simulink model "SixJointFixTimeMode"  (R2019b)
settings: Solver=ode45  StartTime=0.0  StopTime=1  FixedStep=0.01  RelTol=1e-3
values from neighbouring files (symbols this model uses):
  m = [m1;m2;m3;m4;m5;m6]    [SixJointFiniteTimeController.m]    (also in SixJointFixTimeController.m; SixJointFixTimeController2.m; SixJointFixTimeController3.m; SixJointFixTimePlant.m)
  N = N1+N2+N3+N4+N5+N6    [SixJointFiniteTimeController.m]    (also in SixJointFixTimeController.m; SixJointFixTimeController2.m; SixJointFixTimeController3.m; SixJointFixTimePlant.m)
  s = [s1; s2; s3; s4; s5; s6]    [SixJointFiniteTimeController.m]    (also in ctrl2_nijunkang.m = -de + alpha1*abs(-e)^p*sign(-e) + belta1*abs(-e)^E2*sign(-e); ctrl2_test.m = dth + alpha1*abs(th)^p*sign(th) + belta1*abs(th)^E2*sign(th))
undefined symbols (not defined in the file or in its folder): X, Y, Z
libraries: sm_lib x22, nesl_utility x19
settings Model: Creator=user  LastModifiedBy=xyh
settings SolverCC: AlgebraicLoopSolver=LineSearch
settings DataIOCC: ReturnWorkspaceOutputs=off

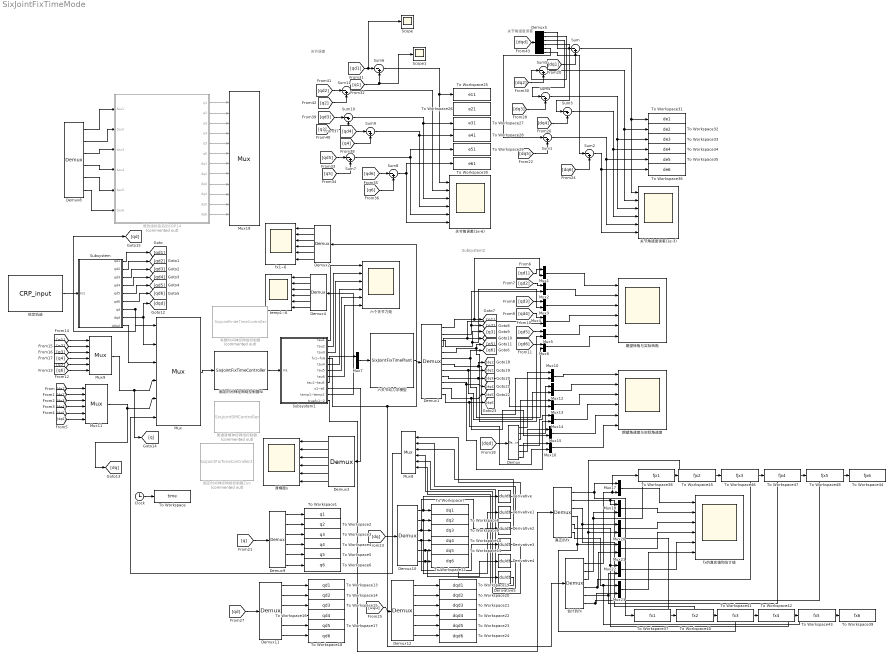
== system SixJointFixTimeMode ==
  note: 关节误差
  note: 关节角速度误差
  note: Subsystem2
  Clock : Clock
  Demux{,2..5,8..12} (10 alike) : Demux  Outputs=6
  Demux1 : Demux  Outputs=12
  Derivative{,1..5} (6 alike) : Derivative
  Mux{,8..9,11} (4 alike) : Mux  Inputs=6
  Mux{1..7,10,12..18,20..23} (19 alike) : Mux  Inputs=2
  Mux19 : Mux  Inputs=12
  Scope : Scope
  Scope1 : Scope
  Subsystem : Subsystem  TreatAsAtomicUnit=on
  Subsystem1 : Subsystem
  Sum{,1..11} (12 alike) : Sum  Inputs=|-+
  To Workspace : ToWorkspace  VariableName=time  SaveFormat=Timeseries  SampleTime=-1
  To Workspace1 : ToWorkspace  VariableName=q1  SaveFormat=Timeseries  SampleTime=-1
  To Workspace10 : ToWorkspace  VariableName=dq4  SaveFormat=Timeseries  SampleTime=-1
  To Workspace11 : ToWorkspace  VariableName=dq5  SaveFormat=Timeseries  SampleTime=-1
  To Workspace12 : ToWorkspace  VariableName=dq6  SaveFormat=Timeseries  SampleTime=-1
  To Workspace13 : ToWorkspace  VariableName=qd1  SaveFormat=Timeseries  SampleTime=-1
  To Workspace14 : ToWorkspace  VariableName=qd2  SaveFormat=Timeseries  SampleTime=-1
  To Workspace15 : ToWorkspace  VariableName=qd3  SaveFormat=Timeseries  SampleTime=-1
  To Workspace16 : ToWorkspace  VariableName=qd4  SaveFormat=Timeseries  SampleTime=-1
  To Workspace17 : ToWorkspace  VariableName=qd5  SaveFormat=Timeseries  SampleTime=-1
  To Workspace18 : ToWorkspace  VariableName=qd6  SaveFormat=Timeseries  SampleTime=-1
  To Workspace19 : ToWorkspace  VariableName=dqd1  SaveFormat=Timeseries  SampleTime=-1
  To Workspace2 : ToWorkspace  VariableName=q2  SaveFormat=Timeseries  SampleTime=-1
  To Workspace20 : ToWorkspace  VariableName=dqd2  SaveFormat=Timeseries  SampleTime=-1
  To Workspace21 : ToWorkspace  VariableName=dqd3  SaveFormat=Timeseries  SampleTime=-1
  To Workspace22 : ToWorkspace  VariableName=dqd4  SaveFormat=Timeseries  SampleTime=-1
  To Workspace23 : ToWorkspace  VariableName=dqd5  SaveFormat=Timeseries  SampleTime=-1
  To Workspace24 : ToWorkspace  VariableName=dqd6  SaveFormat=Timeseries  SampleTime=-1
  To Workspace25 : ToWorkspace  VariableName=e11  SaveFormat=Timeseries  SampleTime=-1
  To Workspace26 : ToWorkspace  VariableName=e21  SaveFormat=Timeseries  SampleTime=-1
  To Workspace27 : ToWorkspace  VariableName=e31  SaveFormat=Timeseries  SampleTime=-1
  To Workspace28 : ToWorkspace  VariableName=e41  SaveFormat=Timeseries  SampleTime=-1
  To Workspace29 : ToWorkspace  VariableName=e51  SaveFormat=Timeseries  SampleTime=-1
  To Workspace3 : ToWorkspace  VariableName=q3  SaveFormat=Timeseries  SampleTime=-1
  To Workspace30 : ToWorkspace  VariableName=e61  SaveFormat=Timeseries  SampleTime=-1
  To Workspace31 : ToWorkspace  VariableName=de1  SaveFormat=Timeseries  SampleTime=-1
  To Workspace32 : ToWorkspace  VariableName=de2  SaveFormat=Timeseries  SampleTime=-1
  To Workspace33 : ToWorkspace  VariableName=de3  SaveFormat=Timeseries  SampleTime=-1
  To Workspace34 : ToWorkspace  VariableName=de4  SaveFormat=Timeseries  SampleTime=-1
  To Workspace35 : ToWorkspace  VariableName=de5  SaveFormat=Timeseries  SampleTime=-1
  To Workspace36 : ToWorkspace  VariableName=de6  SaveFormat=Timeseries  SampleTime=-1
  To Workspace37 : ToWorkspace  VariableName=fx1  SaveFormat=Timeseries  SampleTime=-1
  To Workspace38 : ToWorkspace  VariableName=fjx1  SaveFormat=Timeseries  SampleTime=-1
  To Workspace39 : ToWorkspace  VariableName=fx6  SaveFormat=Timeseries  SampleTime=-1
  To Workspace4 : ToWorkspace  VariableName=q4  SaveFormat=Timeseries  SampleTime=-1
  To Workspace40 : ToWorkspace  VariableName=fx2  SaveFormat=Timeseries  SampleTime=-1
  To Workspace41 : ToWorkspace  VariableName=fx3  SaveFormat=Timeseries  SampleTime=-1
  To Workspace42 : ToWorkspace  VariableName=fx4  SaveFormat=Timeseries  SampleTime=-1
  To Workspace43 : ToWorkspace  VariableName=fx5  SaveFormat=Timeseries  SampleTime=-1
  To Workspace44 : ToWorkspace  VariableName=fjx6  SaveFormat=Timeseries  SampleTime=-1
  To Workspace45 : ToWorkspace  VariableName=fjx2  SaveFormat=Timeseries  SampleTime=-1
  To Workspace46 : ToWorkspace  VariableName=fjx3  SaveFormat=Timeseries  SampleTime=-1
  To Workspace47 : ToWorkspace  VariableName=fjx4  SaveFormat=Timeseries  SampleTime=-1
  To Workspace48 : ToWorkspace  VariableName=fjx5  SaveFormat=Timeseries  SampleTime=-1
  To Workspace5 : ToWorkspace  VariableName=q5  SaveFormat=Timeseries  SampleTime=-1
  To Workspace6 : ToWorkspace  VariableName=q6  SaveFormat=Timeseries  SampleTime=-1
  To Workspace7 : ToWorkspace  VariableName=dq1  SaveFormat=Timeseries  SampleTime=-1
  To Workspace8 : ToWorkspace  VariableName=dq2  SaveFormat=Timeseries  SampleTime=-1
  To Workspace9 : ToWorkspace  VariableName=dq3  SaveFormat=Timeseries  SampleTime=-1
  fx1~6 : Scope  NumInputPorts=6
  "fx的真实值和估计值 " : Scope  NumInputPorts=6
  temp1~6 : Scope  NumInputPorts=6
  估计的fx : Demux  Outputs=6
  "修改坐标系后的CRP14 " : Subsystem  Commented=on
      mask Display: image('$imagefile'); % Use "Edit Image" on toolstrip to change.
  六个关节力矩 : Scope  NumInputPorts=6
  "六关节动力学模型 " : S-Function  FunctionName=SixJointFixTimePlant  SFunctionDeploymentMode=off  EnableBusSupport=off
  关节角误差(1e-6) : Scope  NumInputPorts=6
  关节角速度误差(1e-3) : Scope  NumInputPorts=6
  固定时间神经网络控制器Ni : S-Function  FunctionName=SixJointFixTimeController  SFunctionDeploymentMode=off  EnableBusSupport=off
  固定时间神经网络控制器Zuo : S-Function  Commented=on  FunctionName=SixJointFixTimeController2  SFunctionDeploymentMode=off  EnableBusSupport=off
  普通滑模神经网络控制器 : S-Function  Commented=on  FunctionName=SixJointSMController  SFunctionDeploymentMode=off  EnableBusSupport=off
  有限时间神经网络控制器 : S-Function  Commented=on  FunctionName=SixJointFiniteTimeController  SFunctionDeploymentMode=off  EnableBusSupport=off
  期望角速度与实际角速度 : Scope  NumInputPorts=6
  期望转角与实际转角 : Scope  NumInputPorts=6
  滑模面s : Scope  NumInputPorts=6
  真正的fx : Demux  Outputs=6
  给定轨迹 : S-Function  FunctionName=CRP_input  SFunctionDeploymentMode=off  EnableBusSupport=off
  wires:
  Clock/1 -> To Workspace/1
  [dq1] -> Mux11/1
  [dq4] -> Mux11/4
  [dq2] -> Mux11/2
  [dq3] -> Mux11/3
  [dq5] -> Mux11/5
  [dq6] -> Mux11/6
  Demux3/1 -> 滑模面s/1
  Demux3/2 -> 滑模面s/2
  Demux3/3 -> 滑模面s/3
  [q1] -> Mux9/1
  [q2] -> Mux9/2
  [q3] -> Mux9/3
  [q4] -> Mux9/4
  [q5] -> Mux9/5
  [q6] -> Mux9/6
  "六关节动力学模型 "/1 -> Demux1/1
  Mux11/1 -> [dq], Mux/5
  Mux9/1 -> [q], Mux/4
  给定轨迹/1 -> Subsystem/1(In1)
  Subsystem/7(qd) -> [qd], Mux/1
  Subsystem/8(dqd) -> [dqd], Mux/2
  Subsystem/9(ddqd) -> Mux/3
  Subsystem/1(qd1) -> [qd1]
  Subsystem/2(qd2) -> [qd2]
  Subsystem/3(qd3) -> [qd3]
  Subsystem/4(qd4) -> [qd4]
  Subsystem/5(qd5) -> [qd5]
  Subsystem/6(qd6) -> [qd6]
  Sum6/1 -> 关节角误差(1e-6)/1, To Workspace25/1
  Sum11/1 -> 关节角误差(1e-6)/2, To Workspace26/1
  Sum10/1 -> 关节角误差(1e-6)/3, To Workspace27/1
  Sum9/1 -> 关节角误差(1e-6)/4, To Workspace28/1
  Sum7/1 -> To Workspace29/1, 关节角误差(1e-6)/5
  Sum8/1 -> 关节角误差(1e-6)/6, To Workspace30/1
  Mux1/1 -> 期望转角与实际转角/1
  Mux2/1 -> 期望转角与实际转角/2
  Mux3/1 -> 期望转角与实际转角/3
  Mux4/1 -> 期望转角与实际转角/4
  Mux5/1 -> 期望转角与实际转角/5
  Mux6/1 -> 期望转角与实际转角/6
  Mux10/1 -> 期望角速度与实际角速度/1
  Mux12/1 -> 期望角速度与实际角速度/2
  Mux13/1 -> 期望角速度与实际角速度/3
  Mux14/1 -> 期望角速度与实际角速度/4
  Mux15/1 -> 期望角速度与实际角速度/5
  Mux16/1 -> 期望角速度与实际角速度/6
  Demux/4 -> Mux14/1
  Demux1/12 -> Mux16/2, [dq6]
  Demux1/2 -> [q2], Mux2/2
  [qd2] -> Mux2/1
  Demux1/4 -> Mux4/2, [q4]
  [qd1] -> Mux1/1
  Demux/3 -> Mux13/1
  Demux/6 -> Mux16/1
  Demux1/10 -> Mux14/2, [dq4]
  Demux/5 -> Mux15/1
  Demux/1 -> Mux10/1
  Demux1/9 -> Mux13/2, [dq3]
  [dqd] -> Demux/1
  [qd6] -> Mux6/1
  Demux1/7 -> Mux10/2, [dq1]
  [qd3] -> Mux3/1
  Demux1/11 -> [dq5], Mux15/2
  [qd4] -> Mux4/1
  [qd5] -> Mux5/1
  Demux1/5 -> Mux5/2, [q5]
  Demux/2 -> Mux12/1
  Demux1/6 -> [q6], Mux6/2
  Demux1/8 -> Mux12/2, [dq2]
  Demux1/3 -> [q3], Mux3/2
  Sum/1 -> To Workspace31/1, 关节角速度误差(1e-3)/1
  Sum5/1 -> To Workspace32/1, 关节角速度误差(1e-3)/2
  Sum4/1 -> To Workspace33/1, 关节角速度误差(1e-3)/3
  Sum3/1 -> 关节角速度误差(1e-3)/4, To Workspace34/1
  Sum1/1 -> 关节角速度误差(1e-3)/5, To Workspace35/1
  Sum2/1 -> 关节角速度误差(1e-3)/6, To Workspace36/1
  [dq2] -> Sum5/2
  Demux5/4 -> Sum3/1
  Demux5/5 -> Sum1/1
  Demux5/3 -> Sum4/1
  [dq5] -> Sum1/2
  Demux5/1 -> Sum/1
  [dq6] -> Sum2/2
  Demux5/6 -> Sum2/1
  Demux5/2 -> Sum5/1
  [dq3] -> Sum4/2
  [dq4] -> Sum3/2
  [dq1] -> Sum/2
  [q5] -> Sum7/2
  [qd1] -> Scope/1, Sum6/1
  [qd2] -> Sum11/1
  [q4] -> Sum9/2
  [qd3] -> Sum10/1
  [qd4] -> Sum9/1
  [q3] -> Sum10/2
  [qd5] -> Sum7/1
  [q6] -> Sum8/2
  [qd6] -> Sum8/1
  [q2] -> Sum11/2
  [q1] -> Scope1/1, Sum6/2
  [dqd] -> Demux5/1
  Mux/1 -> 固定时间神经网络控制器Ni/1
  Demux3/4 -> 滑模面s/4
  Demux3/5 -> 滑模面s/5
  Demux3/6 -> 滑模面s/6
  Demux2/1 -> fx1~6/1
  Demux2/2 -> fx1~6/2
  Demux2/3 -> fx1~6/3
  Demux2/4 -> fx1~6/4
  Demux2/5 -> fx1~6/5
  Demux2/6 -> fx1~6/6
  "修改坐标系后的CRP14 "/1(q1) -> Mux19/1
  "修改坐标系后的CRP14 "/2(q2) -> Mux19/2
  "修改坐标系后的CRP14 "/3(q3) -> Mux19/3
  "修改坐标系后的CRP14 "/4(q4) -> Mux19/4
  "修改坐标系后的CRP14 "/5(q5) -> Mux19/5
  "修改坐标系后的CRP14 "/6(q6) -> Mux19/6
  "修改坐标系后的CRP14 "/7(dq1) -> Mux19/7
  "修改坐标系后的CRP14 "/8(dq2) -> Mux19/8
  "修改坐标系后的CRP14 "/9(dq3) -> Mux19/9
  "修改坐标系后的CRP14 "/10(dq4) -> Mux19/10
  "修改坐标系后的CRP14 "/11(dq5) -> Mux19/11
  "修改坐标系后的CRP14 "/12(dq6) -> Mux19/12
  Demux8/1 -> "修改坐标系后的CRP14 "/1(tau1)
  Demux8/2 -> "修改坐标系后的CRP14 "/2(tau2)
  Demux8/3 -> "修改坐标系后的CRP14 "/3(tau3)
  Demux8/4 -> "修改坐标系后的CRP14 "/4(tau4)
  Demux8/5 -> "修改坐标系后的CRP14 "/5(tau5)
  Demux8/6 -> "修改坐标系后的CRP14 "/6(tau6)
  固定时间神经网络控制器Ni/1 -> Subsystem1/1(In1)
  Subsystem1/1(tau1) -> 六个关节力矩/1
  Subsystem1/2(tau2) -> 六个关节力矩/2
  Subsystem1/3(tau3) -> 六个关节力矩/3
  Subsystem1/5(tau4) -> 六个关节力矩/4
  Subsystem1/6(tau5) -> 六个关节力矩/5
  Subsystem1/7(tau6) -> 六个关节力矩/6
  Subsystem1/9(s1~s6) -> Demux3/1
  Subsystem1/4(fx1~fx6) -> Demux2/1, 估计的fx/1
  Subsystem1/8(tau1~tau6) -> Mux7/1
  Demux4/6 -> temp1~6/6
  Demux4/5 -> temp1~6/5
  Demux4/4 -> temp1~6/4
  Demux4/3 -> temp1~6/3
  Demux4/2 -> temp1~6/2
  Demux4/1 -> temp1~6/1
  Subsystem1/10(temp1~temp1) -> Demux4/1
  Mux7/1 -> "六关节动力学模型 "/1
  [q] -> Demux9/1
  [dq] -> Demux10/1
  [qd] -> Demux11/1
  [dqd] -> Demux12/1
  Demux11/1 -> To Workspace13/1
  Demux11/2 -> To Workspace14/1
  Demux11/3 -> To Workspace15/1
  Demux11/4 -> To Workspace16/1
  Demux11/5 -> To Workspace17/1
  Demux11/6 -> To Workspace18/1
  Demux12/1 -> To Workspace19/1
  Demux12/2 -> To Workspace20/1
  Demux12/3 -> To Workspace21/1
  Demux12/4 -> To Workspace22/1
  Demux12/5 -> To Workspace23/1
  Demux12/6 -> To Workspace24/1
  Demux9/1 -> To Workspace1/1
  Demux9/2 -> To Workspace2/1
  Demux9/3 -> To Workspace3/1
  Demux9/4 -> To Workspace4/1
  Demux9/5 -> To Workspace5/1
  Demux9/6 -> To Workspace6/1
  Demux10/1 -> Derivative/1, To Workspace7/1
  Demux10/2 -> Derivative1/1, To Workspace8/1
  Demux10/3 -> Derivative2/1, To Workspace9/1
  Demux10/4 -> Derivative3/1, To Workspace10/1
  Demux10/5 -> Derivative4/1, To Workspace11/1
  Demux10/6 -> Derivative5/1, To Workspace12/1
  Demux1/1 -> [q1], Mux1/2
  Derivative/1 -> Mux8/1
  Derivative1/1 -> Mux8/2
  Derivative2/1 -> Mux8/3
  Derivative3/1 -> Mux8/4
  Derivative4/1 -> Mux8/5
  Derivative5/1 -> Mux8/6
  Mux8/1 -> Mux/6
  Subsystem1/11(truefx1~2) -> 真正的fx/1
  真正的fx/1 -> Mux17/1, To Workspace37/1
  估计的fx/1 -> To Workspace38/1, Mux17/2
  真正的fx/2 -> To Workspace40/1, Mux18/1
  估计的fx/2 -> Mux18/2, To Workspace45/1
  真正的fx/3 -> To Workspace41/1, Mux20/1
  估计的fx/3 -> To Workspace46/1, Mux20/2
  真正的fx/4 -> To Workspace42/1, Mux21/1
  估计的fx/4 -> To Workspace47/1, Mux21/2
  真正的fx/5 -> To Workspace43/1, Mux22/1
  估计的fx/5 -> To Workspace48/1, Mux22/2
  真正的fx/6 -> To Workspace39/1, Mux23/1
  估计的fx/6 -> To Workspace44/1, Mux23/2
  Mux17/1 -> "fx的真实值和估计值 "/1
  Mux18/1 -> "fx的真实值和估计值 "/2
  Mux20/1 -> "fx的真实值和估计值 "/3
  Mux21/1 -> "fx的真实值和估计值 "/4
  Mux22/1 -> "fx的真实值和估计值 "/5
  Mux23/1 -> "fx的真实值和估计值 "/6

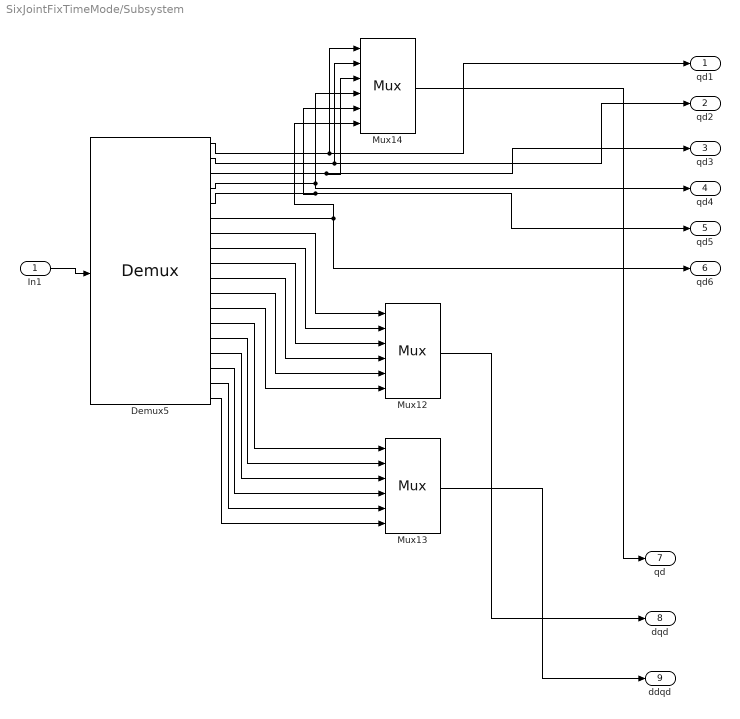
== system SixJointFixTimeMode/Subsystem ==
  In1 : Inport
  Demux5 : Demux  Outputs=18
  Mux12 : Mux  Inputs=6
  Mux13 : Mux  Inputs=6
  Mux14 : Mux  Inputs=6
  qd1 : Outport
  qd2 : Outport  Port=2
  qd3 : Outport  Port=3
  qd4 : Outport  Port=4
  qd5 : Outport  Port=5
  qd6 : Outport  Port=6
  qd : Outport  Port=7
  dqd : Outport  Port=8
  ddqd : Outport  Port=9
  wires:
  Demux5/8 -> Mux12/2
  Demux5/2 -> Mux14/2, qd2/1
  Demux5/3 -> Mux14/3, qd3/1
  Mux13/1 -> ddqd/1
  Demux5/11 -> Mux12/5
  Demux5/4 -> qd4/1, Mux14/4
  Demux5/1 -> Mux14/1, qd1/1
  Demux5/5 -> Mux14/5, qd5/1
  Demux5/13 -> Mux13/1
  In1/1 -> Demux5/1
  Demux5/7 -> Mux12/1
  Demux5/6 -> Mux14/6, qd6/1
  Mux12/1 -> dqd/1
  Demux5/12 -> Mux12/6
  Demux5/14 -> Mux13/2
  Demux5/18 -> Mux13/6
  Demux5/16 -> Mux13/4
  Mux14/1 -> qd/1
  Demux5/17 -> Mux13/5
  Demux5/10 -> Mux12/4
  Demux5/9 -> Mux12/3
  Demux5/15 -> Mux13/3

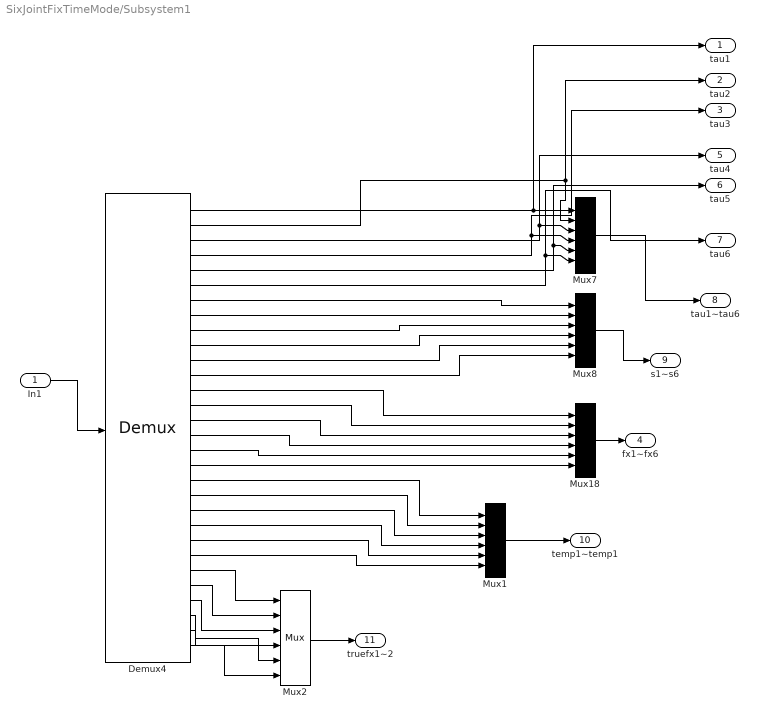
== system SixJointFixTimeMode/Subsystem1 ==
  In1 : Inport
  Demux4 : Demux  Outputs=30
  Mux{1..2,7..8,18} (5 alike) : Mux  Inputs=6
  tau1 : Outport
  tau2 : Outport  Port=2
  tau3 : Outport  Port=3
  fx1~fx6 : Outport  Port=4
  tau4 : Outport  Port=5
  tau5 : Outport  Port=6
  tau6 : Outport  Port=7
  tau1~tau6 : Outport  Port=8
  s1~s6 : Outport  Port=9
  temp1~temp1 : Outport  Port=10
  truefx1~2 : Outport  Port=11
  wires:
  Demux4/7 -> Mux8/1
  Demux4/11 -> Mux8/5
  Mux18/1 -> fx1~fx6/1
  Demux4/5 -> Mux7/5, tau5/1
  Demux4/14 -> Mux18/2
  Demux4/4 -> tau3/1, Mux7/4
  Demux4/13 -> Mux18/1
  Demux4/12 -> Mux8/6
  Demux4/2 -> Mux7/2, tau2/1
  Demux4/16 -> Mux18/4
  Demux4/17 -> Mux18/5
  Demux4/18 -> Mux18/6
  Demux4/10 -> Mux8/4
  Demux4/1 -> tau1/1, Mux7/1
  Demux4/8 -> Mux8/2
  Mux8/1 -> s1~s6/1
  Mux7/1 -> tau1~tau6/1
  Demux4/9 -> Mux8/3
  Demux4/6 -> tau6/1, Mux7/6
  Demux4/3 -> tau4/1, Mux7/3
  Demux4/15 -> Mux18/3
  In1/1 -> Demux4/1
  Demux4/19 -> Mux1/1
  Demux4/20 -> Mux1/2
  Demux4/21 -> Mux1/3
  Demux4/22 -> Mux1/4
  Demux4/23 -> Mux1/5
  Demux4/24 -> Mux1/6
  Mux1/1 -> temp1~temp1/1
  Mux2/1 -> truefx1~2/1
  Demux4/25 -> Mux2/1
  Demux4/26 -> Mux2/2
  Demux4/27 -> Mux2/3
  Demux4/28 -> Mux2/4
  Demux4/29 -> Mux2/5
  Demux4/30 -> Mux2/6

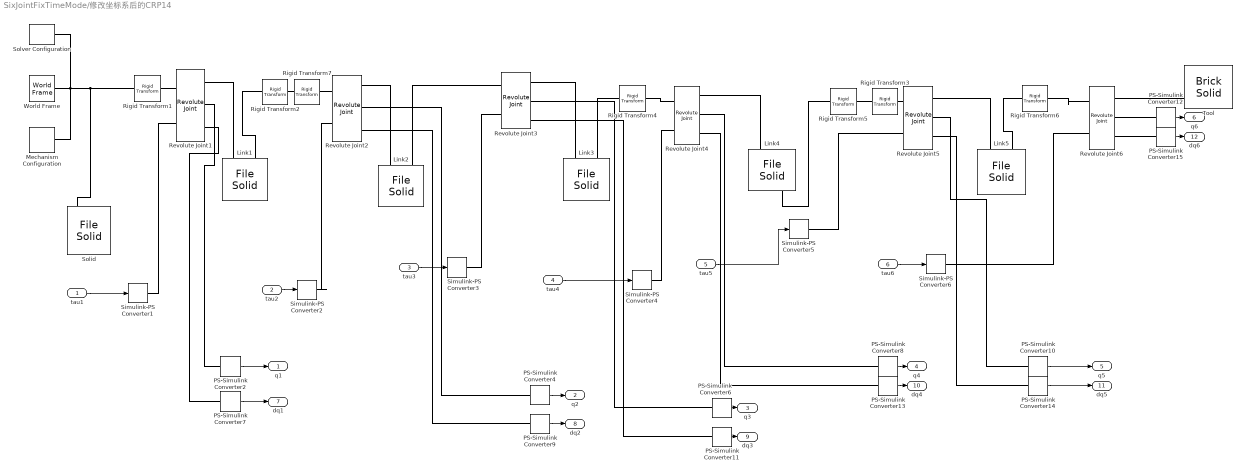
== system SixJointFixTimeMode/修改坐标系后的CRP14  ==
  tau1 : Inport
  tau2 : Inport  Port=2
  tau3 : Inport  Port=3
  tau4 : Inport  Port=4
  tau5 : Inport  Port=5
  tau6 : Inport  Port=6
  Link1 : sm_lib/Body Elements/File Solid  ExtGeomFileName=D:\matlab_course\Manipulator-master\YangHaixinManipulatorSimulator\CR1402 腰部组件-wf_默认_sldprt.STEP  UnitType=FromFile  ExtGeomFileUnits=m  StepReaderType=OCC  ExportEntireGeometry=off  InertiaType=CalculateFromGeometry  Mass=1  MassUnits=kg  CenterOfMass=[0 0 0]  CenterOfMassUnits=m  MomentsOfInertia=[1 1 1]  MomentsOfInertiaUnits=kg*m^2  ProductsOfInertia=[0 0 0]  ProductsOfInertiaUnits=kg*m^2  BasedOnType=Density  Density=1000  DensityUnits=kg/(m^3)  DoExposeReferenceFrame=on  SerializedFrames=<Frames><Frame><Id>Frame1</Id><Value><Name>F1</Name><Origin><Source>GeometricFeature</Source><FeatureName>planar surface 99</FeatureName></Origin><PrimaryAxis><DefinedDirection>+Z</DefinedDirection><Source>ReferenceFrame</Source><SourceDirection>+Z</SourceDirection><FeatureName></FeatureName></PrimaryAxis><SecondaryAxis><DefinedDirection>+X</DefinedDirection><Source>ReferenceFrame</Source><SourceDirection>+X</SourceDirection><FeatureName></FeatureName></SecondaryAxis></Value></Frame><Frame><Id>Frame2</Id><Value><Name>F2</Name><Origin><Source>GeometricFeature</Source><FeatureName>planar surface 124</FeatureName></Origin><PrimaryAxis><DefinedDirection>+Z</DefinedDirection><Source>ReferenceFrame</Source><SourceDirection>+Z</SourceDirection><FeatureName></FeatureName></PrimaryAxis><SecondaryAxis><DefinedDirection>+X</DefinedDirection><Source>ReferenceFrame</Source><SourceDirection>+X</SourceDirection><FeatureName></FeatureName></SecondaryAxis></Value></Frame><Frame><Id>Frame3</Id><Value><Name>Link1CM</Name><Origin><Source>CenterOfMassFrame</Source><FeatureName></FeatureName></Origin><PrimaryAxis><DefinedDirection>+Z</DefinedDirection><Source>CenterOfMassFrame</Source><SourceDirection>+Z</SourceDirection><FeatureName></FeatureName></PrimaryAxis><SecondaryAxis><DefinedDirection>+X</DefinedDirection><Source>CenterOfMassFrame</Source><SourceDirection>+X</SourceDirection><FeatureName></FeatureName></SecondaryAxis></Value></Frame></Frames>  GraphicType=FromGeometry  MarkerShape=Sphere  MarkerSize=10  GraphicVisPropType=SimpleVisualProperties  GraphicDiffuseColor=[153/255 50/255 204/255]  GraphicSpecularColor=[0.5 0.5 0.5 1.0]  GraphicAmbientColor=[0.15 0.15 0.15 1.0]  GraphicEmissiveColor=[0.0 0.0 0.0 1.0]  GraphicShininess=75  GraphicOpacity=1.0
  Link2 : sm_lib/Body Elements/File Solid  ExtGeomFileName=D:\matlab_course\Manipulator-master\YangHaixinManipulatorSimulator\CR1403 大臂组件-wf_默认_sldprt.STEP  UnitType=FromFile  ExtGeomFileUnits=m  StepReaderType=OCC  ExportEntireGeometry=off  InertiaType=CalculateFromGeometry  Mass=1  MassUnits=kg  CenterOfMass=[0 0 0]  CenterOfMassUnits=m  MomentsOfInertia=[1 1 1]  MomentsOfInertiaUnits=kg*m^2  ProductsOfInertia=[0 0 0]  ProductsOfInertiaUnits=kg*m^2  BasedOnType=Density  Density=1000  DensityUnits=kg/(m^3)  DoExposeReferenceFrame=on  SerializedFrames=<Frames><Frame><Id>Frame1</Id><Value><Name>F1</Name><Origin><Source>GeometricFeature</Source><FeatureName>planar surface 28</FeatureName></Origin><PrimaryAxis><DefinedDirection>+Z</DefinedDirection><Source>ReferenceFrame</Source><SourceDirection>-X</SourceDirection><FeatureName></FeatureName></PrimaryAxis><SecondaryAxis><DefinedDirection>+X</DefinedDirection><Source>ReferenceFrame</Source><SourceDirection>+Z</SourceDirection><FeatureName></FeatureName></SecondaryAxis></Value></Frame><Frame><Id>Frame2</Id><Value><Name>F2</Name><Origin><Source>GeometricFeature</Source><FeatureName>planar surface 32</FeatureName></Origin><PrimaryAxis><DefinedDirection>+Z</DefinedDirection><Source>ReferenceFrame</Source><SourceDirection>-X</SourceDirection><FeatureName></FeatureName></PrimaryAxis><SecondaryAxis><DefinedDirection>+X</DefinedDirection><Source>ReferenceFrame</Source><SourceDirection>+Z</SourceDirection><FeatureName></FeatureName></SecondaryAxis></Value></Frame><Frame><Id>Frame3</Id><Value><Name>Link2CM</Name><Origin><Source>CenterOfMassFrame</Source><FeatureName></FeatureName></Origin><PrimaryAxis><DefinedDirection>+Z</DefinedDirection><Source>CenterOfMassFrame</Source><SourceDirection>-X</SourceDirection><FeatureName></FeatureName></PrimaryAxis><SecondaryAxis><DefinedDirection>+X</DefinedDirection><Source>CenterOfMassFrame</Source><SourceDirection>+Z</SourceDirection><FeatureName></FeatureName></SecondaryAxis></Value></Frame></Frames>  GraphicType=FromGeometry  MarkerShape=Sphere  MarkerSize=10  GraphicVisPropType=SimpleVisualProperties  GraphicDiffuseColor=[186/255 85/255 211/255]  GraphicSpecularColor=[0.5 0.5 0.5 1.0]  GraphicAmbientColor=[0.15 0.15 0.15 1.0]  GraphicEmissiveColor=[0.0 0.0 0.0 1.0]  GraphicShininess=75  GraphicOpacity=1.0
  Link3 : sm_lib/Body Elements/File Solid  ExtGeomFileName=D:\matlab_course\Manipulator-master\YangHaixinManipulatorSimulator\CR1404 肘部组件-wf_默认_sldprt.STEP  UnitType=FromFile  ExtGeomFileUnits=m  StepReaderType=OCC  ExportEntireGeometry=off  InertiaType=CalculateFromGeometry  Mass=1  MassUnits=kg  CenterOfMass=[0 0 0]  CenterOfMassUnits=m  MomentsOfInertia=[1 1 1]  MomentsOfInertiaUnits=kg*m^2  ProductsOfInertia=[0 0 0]  ProductsOfInertiaUnits=kg*m^2  BasedOnType=Density  Density=1000  DensityUnits=kg/(m^3)  DoExposeReferenceFrame=on  SerializedFrames=<Frames><Frame><Id>Frame1</Id><Value><Name>F1</Name><Origin><Source>GeometricFeature</Source><FeatureName>planar surface 166</FeatureName></Origin><PrimaryAxis><DefinedDirection>+Z</DefinedDirection><Source>ReferenceFrame</Source><SourceDirection>+Y</SourceDirection><FeatureName></FeatureName></PrimaryAxis><SecondaryAxis><DefinedDirection>+X</DefinedDirection><Source>ReferenceFrame</Source><SourceDirection>+Z</SourceDirection><FeatureName></FeatureName></SecondaryAxis></Value></Frame><Frame><Id>Frame2</Id><Value><Name>F2</Name><Origin><Source>GeometricFeature</Source><FeatureName>planar surface 147</FeatureName></Origin><PrimaryAxis><DefinedDirection>+Z</DefinedDirection><Source>ReferenceFrame</Source><SourceDirection>+Y</SourceDirection><FeatureName></FeatureName></PrimaryAxis><SecondaryAxis><DefinedDirection>+X</DefinedDirection><Source>ReferenceFrame</Source><SourceDirection>+Z</SourceDirection><FeatureName></FeatureName></SecondaryAxis></Value></Frame><Frame><Id>Frame3</Id><Value><Name>Link3CM</Name><Origin><Source>CenterOfMassFrame</Source><FeatureName></FeatureName></Origin><PrimaryAxis><DefinedDirection>+Z</DefinedDirection><Source>CenterOfMassFrame</Source><SourceDirection>+Y</SourceDirection><FeatureName></FeatureName></PrimaryAxis><SecondaryAxis><DefinedDirection>+X</DefinedDirection><Source>CenterOfMassFrame</Source><SourceDirection>+Z</SourceDirection><FeatureName></FeatureName></SecondaryAxis></Value></Frame></Frames>  GraphicType=FromGeometry  MarkerShape=Sphere  MarkerSize=10  GraphicVisPropType=SimpleVisualProperties  GraphicDiffuseColor=[218/225 112/255 214/255]  GraphicSpecularColor=[0.5 0.5 0.5 1.0]  GraphicAmbientColor=[0.15 0.15 0.15 1.0]  GraphicEmissiveColor=[0.0 0.0 0.0 1.0]  GraphicShininess=75  GraphicOpacity=1.0
  Link4 : sm_lib/Body Elements/File Solid  ExtGeomFileName=D:\matlab_course\Manipulator-master\YangHaixinManipulatorSimulator\CR1405 小臂组件-wf_默认_sldprt.STEP  UnitType=FromFile  ExtGeomFileUnits=m  StepReaderType=OCC  ExportEntireGeometry=off  InertiaType=CalculateFromGeometry  Mass=1  MassUnits=kg  CenterOfMass=[0 0 0]  CenterOfMassUnits=m  MomentsOfInertia=[1 1 1]  MomentsOfInertiaUnits=kg*m^2  ProductsOfInertia=[0 0 0]  ProductsOfInertiaUnits=kg*m^2  BasedOnType=Density  Density=1000  DensityUnits=kg/(m^3)  DoExposeReferenceFrame=on  SerializedFrames=<Frames><Frame><Id>Frame1</Id><Value><Name>F1</Name><Origin><Source>GeometricFeature</Source><FeatureName>planar surface 17</FeatureName></Origin><PrimaryAxis><DefinedDirection>+Z</DefinedDirection><Source>ReferenceFrame</Source><SourceDirection>+X</SourceDirection><FeatureName></FeatureName></PrimaryAxis><SecondaryAxis><DefinedDirection>+X</DefinedDirection><Source>ReferenceFrame</Source><SourceDirection>+Z</SourceDirection><FeatureName></FeatureName></SecondaryAxis></Value></Frame><Frame><Id>Frame3</Id><Value><Name>Link4CM</Name><Origin><Source>CenterOfMassFrame</Source><FeatureName></FeatureName></Origin><PrimaryAxis><DefinedDirection>+Z</DefinedDirection><Source>CenterOfMassFrame</Source><SourceDirection>+X</SourceDirection><FeatureName></FeatureName></PrimaryAxis><SecondaryAxis><DefinedDirection>+X</DefinedDirection><Source>CenterOfMassFrame</Source><SourceDirection>+Z</SourceDirection><FeatureName></FeatureName></SecondaryAxis></Value></Frame><Frame><Id>Frame4</Id><Value><Name>F4</Name><Origin><Source>GeometricFeature</Source><FeatureName>circular curve 348</FeatureName></Origin><PrimaryAxis><DefinedDirection>+Z</DefinedDirection><Source>ReferenceFrame</Source><SourceDirection>+X</SourceDirection><FeatureName></FeatureName></PrimaryAxis><SecondaryAxis><DefinedDirection>+X</DefinedDirection><Source>ReferenceFrame</Source><SourceDirection>+Z</SourceDirection><FeatureName></FeatureName></SecondaryAxis></Value></Frame></Frames>  GraphicType=FromGeometry  MarkerShape=Sphere  MarkerSize=10  GraphicVisPropType=SimpleVisualProperties  GraphicDiffuseColor=[221/255 160/255 221/255]  GraphicSpecularColor=[0.5 0.5 0.5 1.0]  GraphicAmbientColor=[0.15 0.15 0.15 1.0]  GraphicEmissiveColor=[0.0 0.0 0.0 1.0]  GraphicShininess=75  GraphicOpacity=1.0
  Link5 : sm_lib/Body Elements/File Solid  ExtGeomFileName=D:\matlab_course\Manipulator-master\YangHaixinManipulatorSimulator\CR1806 腕部组件_默认_sldprt.STEP  UnitType=FromFile  ExtGeomFileUnits=m  StepReaderType=OCC  ExportEntireGeometry=off  InertiaType=CalculateFromGeometry  Mass=1  MassUnits=kg  CenterOfMass=[0 0 0]  CenterOfMassUnits=m  MomentsOfInertia=[1 1 1]  MomentsOfInertiaUnits=kg*m^2  ProductsOfInertia=[0 0 0]  ProductsOfInertiaUnits=kg*m^2  BasedOnType=Density  Density=1000  DensityUnits=kg/(m^3)  DoExposeReferenceFrame=on  SerializedFrames=<Frames><Frame><Id>Frame1</Id><Value><Name>F1</Name><Origin><Source>GeometricFeature</Source><FeatureName>planar surface 10</FeatureName></Origin><PrimaryAxis><DefinedDirection>+X</DefinedDirection><Source>ReferenceFrame</Source><SourceDirection>+Z</SourceDirection><FeatureName></FeatureName></PrimaryAxis><SecondaryAxis><DefinedDirection>+Y</DefinedDirection><Source>ReferenceFrame</Source><SourceDirection>+X</SourceDirection><FeatureName></FeatureName></SecondaryAxis></Value></Frame><Frame><Id>Frame2</Id><Value><Name>F2</Name><Origin><Source>GeometricFeature</Source><FeatureName>planar surface 95</FeatureName></Origin><PrimaryAxis><DefinedDirection>+X</DefinedDirection><Source>ReferenceFrame</Source><SourceDirection>+Z</SourceDirection><FeatureName></FeatureName></PrimaryAxis><SecondaryAxis><DefinedDirection>+Y</DefinedDirection><Source>ReferenceFrame</Source><SourceDirection>+X</SourceDirection><FeatureName></FeatureName></SecondaryAxis></Value></Frame><Frame><Id>Frame3</Id><Value><Name>Link5CM</Name><Origin><Source>CenterOfMassFrame</Source><FeatureName></FeatureName></Origin><PrimaryAxis><DefinedDirection>+X</DefinedDirection><Source>CenterOfMassFrame</Source><SourceDirection>+Z</SourceDirection><FeatureName></FeatureName></PrimaryAxis><SecondaryAxis><DefinedDirection>+Y</DefinedDirection><Source>CenterOfMassFrame</Source><SourceDirection>+X</SourceDirection><FeatureName></FeatureName></SecondaryAxis></Value></Frame></Frames>  GraphicType=FromGeometry  MarkerShape=Sphere  MarkerSize=10  GraphicVisPropType=SimpleVisualProperties  GraphicDiffuseColor=[0.53 0.63 0.63]  GraphicSpecularColor=[0.5 0.5 0.5 1.0]  GraphicAmbientColor=[0.15 0.15 0.15 1.0]  GraphicEmissiveColor=[0.0 0.0 0.0 1.0]  GraphicShininess=75  GraphicOpacity=1.0
  Mechanism Configuration : sm_lib/Utilities/Mechanism Configuration  UniformGravity=Constant  GravityVector=[0 0 -9.80665]  GravityUnits=m/s^2  LinearizationDelta=0.001
  PS-Simulink Converter{2,4,6..15} (12 alike) : nesl_utility/PS-Simulink Converter  PhysicalDomain=network_engine_domain  SubClassName=ps_output  LeftPortType=input  RightPortType=output  PseudoPeriodic=off  Frequencies=[]  Unit=1  AffineConversion=off
  Revolute Joint{1..6} (6 alike) : sm_lib/Joints/Revolute Joint  JointMode=Normal  SenseConstraintForce=off  SenseConstraintForceX=off  SenseConstraintForceY=off  SenseConstraintForceZ=off  SenseConstraintTorque=off  SenseConstraintTorqueX=off  SenseConstraintTorqueY=off  SenseConstraintTorqueZ=off  SenseTotalForce=off  SenseTotalForceX=off  SenseTotalForceY=off  SenseTotalForceZ=off  SenseTotalTorque=off  SenseTotalTorqueX=off  SenseTotalTorqueY=off  SenseTotalTorqueZ=off  CompositeWrenchDir=FollowerOnBase  CompositeWrenchFrame=BaseFrame  EquilibriumPosition=0  EquilibriumPositionUnits=deg  SpringStiffness=0  SpringStiffnessUnits=N*m/deg  DampingCoefficient=0  DampingCoefficientUnits=N*m/(deg/s)  TorqueActuationMode=InputTorque  MotionActuationMode=ComputedMotion  SensePosition=on  SenseVelocity=on  SenseAcceleration=off  SenseTorqueForce=off  SenseLowerLimitTorqueForce=off  SenseUpperLimitTorqueForce=off  LowerLimitSpecify=off  LowerLimitBound=-90  LowerLimitBoundUnits=deg  LowerLimitStiffness=1e4  LowerLimitStiffnessUnits=N*m/deg  LowerLimitDamping=10  LowerLimitDampingUnits=N*m/(deg/s)  LowerLimitTransitionRegionWidth=0.1  LowerLimitTransitionRegionWidthUnits=deg  UpperLimitSpecify=off  UpperLimitBound=90  UpperLimitBoundUnits=deg  UpperLimitStiffness=1e4  UpperLimitStiffnessUnits=N*m/deg  UpperLimitDamping=10  UpperLimitDampingUnits=N*m/(deg/s)  UpperLimitTransitionRegionWidth=0.1  UpperLimitTransitionRegionWidthUnits=deg  PositionTargetSpecify=off  PositionTargetPriority=High  PositionTargetValue=0  PositionTargetValueUnits=deg  VelocityTargetSpecify=off  VelocityTargetPriority=High  VelocityTargetValue=0  VelocityTargetValueUnits=deg/s
  Rigid Transform1 : sm_lib/Frames and Transforms/Rigid Transform  TranslationMethod=None  TranslationStandardOffset=0  TranslationLengthUnit=m  TranslationStandardAxis=+Z  TranslationCartesianOffset=[0 0 0]  TranslationROffset=0  TranslationROffsetUnits=m  TranslationZOffset=0  TranslationZOffsetUnits=m  TranslationThetaOffset=0  TranslationThetaOffsetUnits=deg  RotationMethod=None  RotationAngleUnits=deg  RotationStandardAxis=+Z  RotationAngle=0.0  RotationArbitraryAxis=[0 0 1]  FollAlignAxisA=+X  BaseAlignAxisA=+Y  FollAlignAxisB=+Y  BaseAlignAxisB=+Z  RotationSequenceAxes=FollowerAxes  RotationSequence=XYX  RotationSequenceAngles=[0 0 0]  RotationSequenceAnglesUnits=deg  RotationMatrix=[1 0 0; 0 1 0; 0 0 1]
  Rigid Transform2 : sm_lib/Frames and Transforms/Rigid Transform  TranslationMethod=None  TranslationStandardOffset=0  TranslationLengthUnit=m  TranslationStandardAxis=+Z  TranslationCartesianOffset=[0 0 0]  TranslationROffset=0  TranslationROffsetUnits=m  TranslationZOffset=0  TranslationZOffsetUnits=m  TranslationThetaOffset=0  TranslationThetaOffsetUnits=deg  RotationMethod=StandardAxis  RotationAngleUnits=deg  RotationStandardAxis=+X  RotationAngle=90  RotationArbitraryAxis=[0 0 1]  FollAlignAxisA=+X  BaseAlignAxisA=+Y  FollAlignAxisB=+Y  BaseAlignAxisB=+Z  RotationSequenceAxes=FollowerAxes  RotationSequence=XYX  RotationSequenceAngles=[0 0 0]  RotationSequenceAnglesUnits=deg  RotationMatrix=[1 0 0; 0 1 0; 0 0 1]
  Rigid Transform3 : sm_lib/Frames and Transforms/Rigid Transform  TranslationMethod=None  TranslationStandardOffset=0  TranslationLengthUnit=m  TranslationStandardAxis=+Z  TranslationCartesianOffset=[0 0 0]  TranslationROffset=0  TranslationROffsetUnits=m  TranslationZOffset=0  TranslationZOffsetUnits=m  TranslationThetaOffset=0  TranslationThetaOffsetUnits=deg  RotationMethod=StandardAxis  RotationAngleUnits=deg  RotationStandardAxis=+Z  RotationAngle=90  RotationArbitraryAxis=[0 0 1]  FollAlignAxisA=+X  BaseAlignAxisA=+Y  FollAlignAxisB=+Y  BaseAlignAxisB=+Z  RotationSequenceAxes=FollowerAxes  RotationSequence=XYX  RotationSequenceAngles=[0 0 0]  RotationSequenceAnglesUnits=deg  RotationMatrix=[1 0 0; 0 1 0; 0 0 1]
  Rigid Transform4 : sm_lib/Frames and Transforms/Rigid Transform  TranslationMethod=None  TranslationStandardOffset=0  TranslationLengthUnit=m  TranslationStandardAxis=+Z  TranslationCartesianOffset=[0 0 0]  TranslationROffset=0  TranslationROffsetUnits=m  TranslationZOffset=0  TranslationZOffsetUnits=m  TranslationThetaOffset=0  TranslationThetaOffsetUnits=deg  RotationMethod=StandardAxis  RotationAngleUnits=deg  RotationStandardAxis=+X  RotationAngle=90  RotationArbitraryAxis=[0 0 1]  FollAlignAxisA=+X  BaseAlignAxisA=+Y  FollAlignAxisB=+Y  BaseAlignAxisB=+Z  RotationSequenceAxes=FollowerAxes  RotationSequence=XYX  RotationSequenceAngles=[0 0 0]  RotationSequenceAnglesUnits=deg  RotationMatrix=[1 0 0; 0 1 0; 0 0 1]
  Rigid Transform5 : sm_lib/Frames and Transforms/Rigid Transform  TranslationMethod=None  TranslationStandardOffset=0  TranslationLengthUnit=m  TranslationStandardAxis=+Z  TranslationCartesianOffset=[0 0 0]  TranslationROffset=0  TranslationROffsetUnits=m  TranslationZOffset=0  TranslationZOffsetUnits=m  TranslationThetaOffset=0  TranslationThetaOffsetUnits=deg  RotationMethod=StandardAxis  RotationAngleUnits=deg  RotationStandardAxis=+X  RotationAngle=90  RotationArbitraryAxis=[0 0 1]  FollAlignAxisA=+X  BaseAlignAxisA=+Y  FollAlignAxisB=+Y  BaseAlignAxisB=+Z  RotationSequenceAxes=FollowerAxes  RotationSequence=XYX  RotationSequenceAngles=[0 0 0]  RotationSequenceAnglesUnits=deg  RotationMatrix=[1 0 0; 0 1 0; 0 0 1]
  Rigid Transform6 : sm_lib/Frames and Transforms/Rigid Transform  TranslationMethod=None  TranslationStandardOffset=0  TranslationLengthUnit=m  TranslationStandardAxis=+Z  TranslationCartesianOffset=[0 0 0]  TranslationROffset=0  TranslationROffsetUnits=m  TranslationZOffset=0  TranslationZOffsetUnits=m  TranslationThetaOffset=0  TranslationThetaOffsetUnits=deg  RotationMethod=StandardAxis  RotationAngleUnits=deg  RotationStandardAxis=+X  RotationAngle=-90  RotationArbitraryAxis=[0 0 1]  FollAlignAxisA=+X  BaseAlignAxisA=+Y  FollAlignAxisB=+Y  BaseAlignAxisB=+Z  RotationSequenceAxes=FollowerAxes  RotationSequence=XYX  RotationSequenceAngles=[0 0 0]  RotationSequenceAnglesUnits=deg  RotationMatrix=[1 0 0; 0 1 0; 0 0 1]
  Rigid Transform7 : sm_lib/Frames and Transforms/Rigid Transform  TranslationMethod=None  TranslationStandardOffset=0  TranslationLengthUnit=m  TranslationStandardAxis=+Z  TranslationCartesianOffset=[0 0 0]  TranslationROffset=0  TranslationROffsetUnits=m  TranslationZOffset=0  TranslationZOffsetUnits=m  TranslationThetaOffset=0  TranslationThetaOffsetUnits=deg  RotationMethod=StandardAxis  RotationAngleUnits=deg  RotationStandardAxis=+Z  RotationAngle=90  RotationArbitraryAxis=[0 0 1]  FollAlignAxisA=+X  BaseAlignAxisA=+Y  FollAlignAxisB=+Y  BaseAlignAxisB=+Z  RotationSequenceAxes=FollowerAxes  RotationSequence=XYX  RotationSequenceAngles=[0 0 0]  RotationSequenceAnglesUnits=deg  RotationMatrix=[1 0 0; 0 1 0; 0 0 1]
  Simulink-PS Converter{1..6} (6 alike) : nesl_utility/Simulink-PS Converter  PhysicalDomain=network_engine_domain  SubClassName=ps_input  LeftPortType=input  RightPortType=output  PseudoPeriodic=off  Frequencies=[]  NoiseDistribution=none  NoiseParameters=[]  Unit=1  AffineConversion=off  FilteringAndDerivatives=filter  SimscapeFilterOrder=2  InputFilterTimeConstant=0.001  UdotUserProvided=1
  Solid : sm_lib/Body Elements/File Solid  ExtGeomFileName=D:\matlab_course\Manipulator-master\YangHaixinManipulatorSimulator\CR1401 底座组件3-wf_默认_sldprt.STEP  UnitType=FromFile  ExtGeomFileUnits=m  StepReaderType=OCC  ExportEntireGeometry=off  InertiaType=CalculateFromGeometry  Mass=1  MassUnits=kg  CenterOfMass=[0 0 0]  CenterOfMassUnits=m  MomentsOfInertia=[1 1 1]  MomentsOfInertiaUnits=kg*m^2  ProductsOfInertia=[0 0 0]  ProductsOfInertiaUnits=kg*m^2  BasedOnType=Density  Density=1000  DensityUnits=kg/(m^3)  DoExposeReferenceFrame=on  SerializedFrames=<Frames><Frame><Id>Frame1</Id><Value><Name>F1</Name><Origin><Source>GeometricFeature</Source><FeatureName>planar surface 39</FeatureName></Origin><PrimaryAxis><DefinedDirection>+Z</DefinedDirection><Source>ReferenceFrame</Source><SourceDirection>+Z</SourceDirection><FeatureName></FeatureName></PrimaryAxis><SecondaryAxis><DefinedDirection>-X</DefinedDirection><Source>ReferenceFrame</Source><SourceDirection>+X</SourceDirection><FeatureName></FeatureName></SecondaryAxis></Value></Frame><Frame><Id>Frame2</Id><Value><Name>SolidCM</Name><Origin><Source>CenterOfMassFrame</Source><FeatureName></FeatureName></Origin><PrimaryAxis><DefinedDirection>+Z</DefinedDirection><Source>CenterOfMassFrame</Source><SourceDirection>+Z</SourceDirection><FeatureName></FeatureName></PrimaryAxis><SecondaryAxis><DefinedDirection>-X</DefinedDirection><Source>CenterOfMassFrame</Source><SourceDirection>+X</SourceDirection><FeatureName></FeatureName></SecondaryAxis></Value></Frame></Frames>  GraphicType=FromGeometry  MarkerShape=Sphere  MarkerSize=10  GraphicVisPropType=SimpleVisualProperties  GraphicDiffuseColor=[148/255 0 211/255]  GraphicSpecularColor=[0.5 0.5 0.5 1.0]  GraphicAmbientColor=[0.15 0.15 0.15 1.0]  GraphicEmissiveColor=[0.0 0.0 0.0 1.0]  GraphicShininess=75  GraphicOpacity=1.0
      settings: AttributesFormatString=m =%<Mass>%<MassUnits>
  Solver Configuration : nesl_utility/Solver Configuration  PhysicalDomain=network_engine_domain  SubClassName=solver  LeftPortType=input  RightPortType=generic  Tones=[]  Harmonics=[]  SimulateNoise=off  Profile=off  UseLocalSampling=off  EnableSwitchedLinearOptims=on  FrequencyDomain=off  UseCCode=off  RelTol=0.001  AbsTol=1e-06  MinStep=1e-09  ToWorkspace=off  RevertToSquareIcSolve=off  NumHomotopyIterations=100  PhasorMode=off  PhasorModeNumHarmonics=1  DoDC=off  ResidualTolerance=1e-09  UseLocalSolver=off  LocalSolverChoice=NE_BACKWARD_EULER_ADVANCER  LocalSolverSampleTime=0.001  DoFixedCost=off  MaxNonlinIter=3  MaxModeIter=2  LinearAlgebra=Sparse  EquationFormulation=NE_TIME_EF  DelaysMemoryBudget=1024  AutomaticFiltering=on  FilteringTimeConstant=0.001  PartitionStorageMethod=AS_NEEDED  PartitionMemoryBudget=1024  PartitionMethod=FAST
  Tool : sm_lib/Body Elements/Brick Solid  GraphicAmbientColor=[0.15 0.15 0.15 1.0]  BasedOnType=Mass  BrickDimensions=[0.1 0.1 0.1]  BrickDimensionUnits=m  CenterOfMass=[0 0 0]  CenterOfMassUnits=m  GraphicDiffuseColor=[0.0 0.8 1.0]  Density=1000  DensityUnits=kg/(m^3)  DoExposeReferenceFrame=on  GraphicEmissiveColor=[0.0 0.0 0.0 1.0]  ExportEntireGeometry=off  SerializedFrames=<Frames><Frame><Id>Frame2</Id><Value><Name>ToolCM</Name><Origin><Source>CenterOfMassFrame</Source><FeatureName></FeatureName></Origin><PrimaryAxis><DefinedDirection>+Z</DefinedDirection><Source>CenterOfMassFrame</Source><SourceDirection>-Z</SourceDirection><FeatureName></FeatureName></PrimaryAxis><SecondaryAxis><DefinedDirection>+X</DefinedDirection><Source>CenterOfMassFrame</Source><SourceDirection>-X</SourceDirection><FeatureName></FeatureName></SecondaryAxis></Value></Frame><Frame><Id>Frame3</Id><Value><Name>F3</Name><Origin><Source>GeometricFeature</Source><FeatureName>+z surface</FeatureName></Origin><PrimaryAxis><DefinedDirection>+Z</DefinedDirection><Source>ReferenceFrame</Source><SourceDirection>-Z</SourceDirection><FeatureName></FeatureName></PrimaryAxis><SecondaryAxis><DefinedDirection>+X</DefinedDirection><Source>ReferenceFrame</Source><SourceDirection>-X</SourceDirection><FeatureName></FeatureName></SecondaryAxis></Value></Frame></Frames>  MarkerShape=Sphere  MarkerSize=10  GraphicType=FromGeometry  InertiaType=CalculateFromGeometry  Mass=20  MassUnits=kg  MomentsOfInertia=[1 1 1]  MomentsOfInertiaUnits=kg*m^2  GraphicOpacity=1.0  ProductsOfInertia=[0 0 0]  ProductsOfInertiaUnits=kg*m^2  GraphicShininess=75  GraphicSpecularColor=[0.5 0.5 0.5 1.0]  GraphicVisPropType=SimpleVisualProperties
  World Frame : sm_lib/Frames and Transforms/World Frame
  q1 : Outport
  q2 : Outport  Port=2
  q3 : Outport  Port=3
  q4 : Outport  Port=4
  q5 : Outport  Port=5
  q6 : Outport  Port=6
  dq1 : Outport  Port=7
  dq2 : Outport  Port=8
  dq3 : Outport  Port=9
  dq4 : Outport  Port=10
  dq5 : Outport  Port=11
  dq6 : Outport  Port=12
  wires:
  tau1/1 -> Simulink-PS Converter1/1
  tau2/1 -> Simulink-PS Converter2/1
  tau3/1 -> Simulink-PS Converter3/1
  tau4/1 -> Simulink-PS Converter4/1
  tau5/1 -> Simulink-PS Converter5/1
  tau6/1 -> Simulink-PS Converter6/1
  PS-Simulink Converter10/1 -> q5/1
  PS-Simulink Converter2/1 -> q1/1
  PS-Simulink Converter4/1 -> q2/1
  PS-Simulink Converter8/1 -> q4/1
  PS-Simulink Converter12/1 -> q6/1
  PS-Simulink Converter6/1 -> q3/1
  PS-Simulink Converter9/1 -> dq2/1
  PS-Simulink Converter11/1 -> dq3/1
  PS-Simulink Converter13/1 -> dq4/1
  PS-Simulink Converter15/1 -> dq6/1
  PS-Simulink Converter7/1 -> dq1/1
  PS-Simulink Converter14/1 -> dq5/1
  connections:
  Mechanism Configuration/RConn1 -- Rigid Transform1/LConn1 -- Solid/LConn1 -- World Frame/RConn1 -- Solver Configuration/RConn1
  Simulink-PS Converter6/RConn1 -- Revolute Joint6/LConn2
  Revolute Joint4/LConn1 -- Rigid Transform4/RConn1
  Rigid Transform6/RConn1 -- Revolute Joint6/LConn1
  Link4/LConn1 -- Revolute Joint4/RConn1
  Revolute Joint3/RConn1 -- Link3/LConn1
  Revolute Joint3/LConn1 -- Link2/LConn2
  Link2/LConn1 -- Revolute Joint2/RConn1
  Rigid Transform5/LConn1 -- Link4/RConn2
  Rigid Transform5/RConn1 -- Rigid Transform3/LConn1
  Revolute Joint1/LConn1 -- Rigid Transform1/RConn1
  Link1/LConn1 -- Revolute Joint1/RConn1
  Link1/LConn2 -- Rigid Transform2/LConn1
  Rigid Transform4/LConn1 -- Link3/LConn2
  Revolute Joint6/RConn2 -- PS-Simulink Converter12/LConn1
  Link5/LConn2 -- Rigid Transform6/LConn1
  PS-Simulink Converter10/LConn1 -- Revolute Joint5/RConn2
  Revolute Joint1/RConn2 -- PS-Simulink Converter2/LConn1
  PS-Simulink Converter6/LConn1 -- Revolute Joint3/RConn2
  Simulink-PS Converter3/RConn1 -- Revolute Joint3/LConn2
  Revolute Joint2/RConn2 -- PS-Simulink Converter4/LConn1
  Simulink-PS Converter5/RConn1 -- Revolute Joint5/LConn2
  Simulink-PS Converter2/RConn1 -- Revolute Joint2/LConn2
  Simulink-PS Converter4/RConn1 -- Revolute Joint4/LConn2
  PS-Simulink Converter8/LConn1 -- Revolute Joint4/RConn2
  Simulink-PS Converter1/RConn1 -- Revolute Joint1/LConn2
  Revolute Joint6/RConn1 -- Tool/LConn2
  Rigid Transform7/LConn1 -- Rigid Transform2/RConn1
  Rigid Transform7/RConn1 -- Revolute Joint2/LConn1
  Rigid Transform3/RConn1 -- Revolute Joint5/LConn1
  Link5/LConn1 -- Revolute Joint5/RConn1
  Revolute Joint1/RConn3 -- PS-Simulink Converter7/LConn1
  Revolute Joint2/RConn3 -- PS-Simulink Converter9/LConn1
  Revolute Joint3/RConn3 -- PS-Simulink Converter11/LConn1
  Revolute Joint4/RConn3 -- PS-Simulink Converter13/LConn1
  Revolute Joint5/RConn3 -- PS-Simulink Converter14/LConn1
  Revolute Joint6/RConn3 -- PS-Simulink Converter15/LConn1
